simulink model "自动化214呙凯锋202121724408"  (R2023b)
settings: Solver=VariableStepAuto  StartTime=0.0  StopTime=100  RelTol=1e-3
settings Model: Creator=ASUS  LastModifiedBy=ASUS

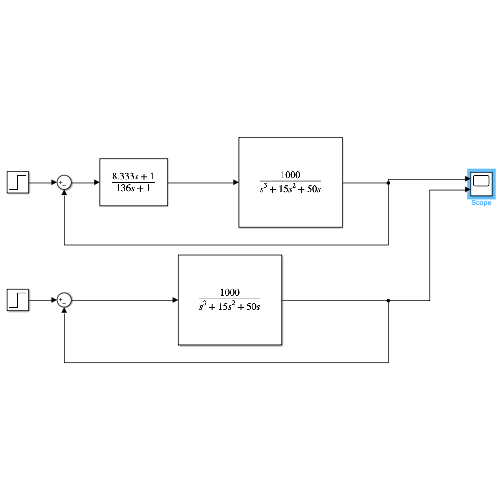
[thumbnail: Simulink's stored preview of the top-level diagram]
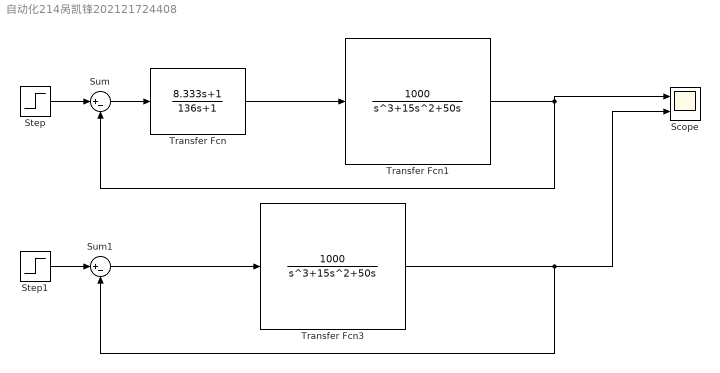
== system 自动化214呙凯锋202121724408 ==
  Scope : Scope  NumInputPorts=2
  Step : Step  SampleTime=0
  Step1 : Step  SampleTime=0
  Sum : Sum  Inputs=|+-
  Sum1 : Sum  Inputs=|+-
  Transfer Fcn : TransferFcn  Numerator=[8.333 1]  Denominator=[136 1]
  Transfer Fcn1 : TransferFcn  Numerator=[ 1000]  Denominator=[1 15 50 0]
  Transfer Fcn3 : TransferFcn  Numerator=[ 1000]  Denominator=[1 15 50 0]
  wires:
  Transfer Fcn/1 -> Transfer Fcn1/1
  Transfer Fcn1/1 -> Sum/2, Scope/1
  Step/1 -> Sum/1
  Sum/1 -> Transfer Fcn/1
  Transfer Fcn3/1 -> Scope/2, Sum1/2
  Sum1/1 -> Transfer Fcn3/1
  Step1/1 -> Sum1/1
